simulink model "interpolation_nD_TestGen62"  (R2017b)
settings: Solver=FixedStepDiscrete  StartTime=0.0  StopTime=10.0  RelTol=1e-3
settings Model: Creator=ktrinh  LastModifiedBy=ktrinh
settings DebuggingCC: ParameterOverflowMsg=none

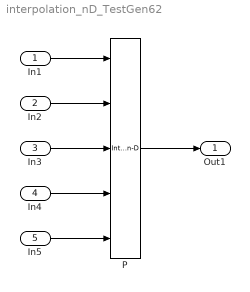
== system interpolation_nD_TestGen62 ==
  In1 : Inport  OutMax=2
  In2 : Inport  Port=2  OutMax=5
  In3 : Inport  Port=3  OutMax=3
  In4 : Inport  Port=4  OutMin=0  OutMax=2
  In5 : Inport  Port=5  PortDimensions=[2 5 3 2]
  P : Interpolation_n-D  NumberOfTableDimensions=4  TableSource=Input port  InterpMethod=Nearest  RequireIndexFractionAsBus=on  NumSelectionDims=4  OutDataTypeStr=double  InternalRulePriority=Speed  RndMeth=Zero  IntermediateResultsDataTypeStr=int32
      settings: InputPortMap=u0,u1,u2,u3,p2
  Out1 : Outport
  wires:
  In1/1 -> P/1
  In2/1 -> P/2
  In3/1 -> P/3
  In4/1 -> P/4
  In5/1 -> P/5
  P/1 -> Out1/1
